simulink model "pid_2"  (Simulink 8.3)
settings: Solver=ode45  StartTime=0.0  StopTime=15  RelTol=1e-3
values from neighbouring files (symbols this model uses):
  Kc = (1.2*tau)/(K*td)    [pid2.m]    (also in pid2.mat = 2.07538801239)
  Kc1 = 0.33*Ku    [pid2.m]    (also in pid2.mat = 3.52049795251)
  Td = 0.5*td    [pid2.m]    (also in pid2.mat = 0.341127043943)
  Td1 = 0.333*Tu    [pid2.m]    (also in pid2.mat = 0.603957217903)
  Ti = 2*td    [pid2.m]    (also in pid2.mat = 1.36450817577)
  Ti1 = 0.5*Tu    [pid2.m]    (also in pid2.mat = 0.906842669523)
libraries: simulink x1
settings Model: Creator=IvanBurgos  LastModifiedBy=IvanBurgos
settings DataIOCC: SignalLoggingSaveFormat=Dataset
settings DebuggingCC: UnderspecifiedInitializationDetection=Simplified  StateNameClashWarn=none
settings GRTTargetCC: CombineOutputUpdateFcns=on  GRTInterface=off

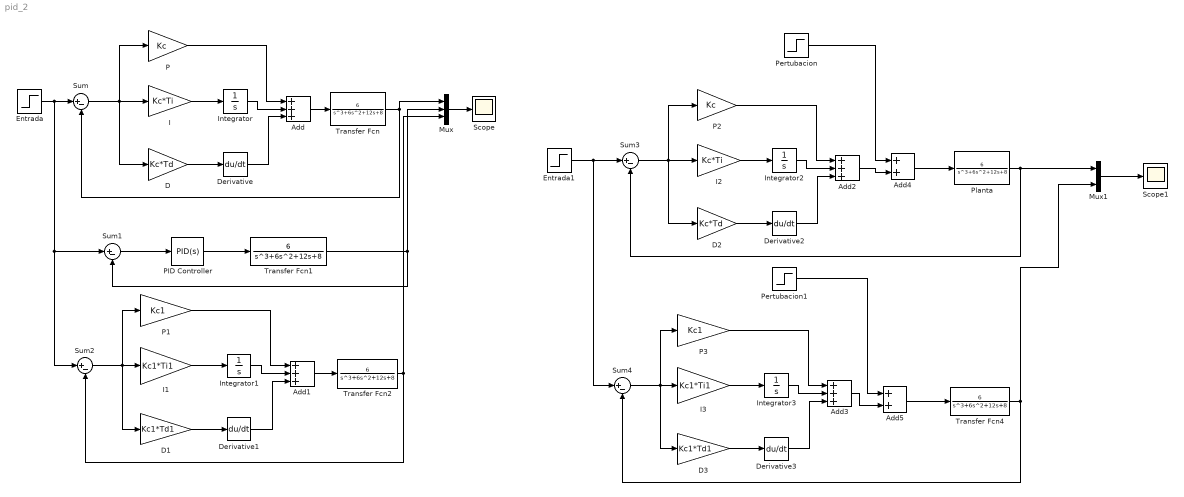
== system pid_2 ==
  Add{,1..3} (4 alike) : Sum  Inputs=+++
  Add4 : Sum
  Add5 : Sum
  D : Gain  Gain=Kc*Td
  D1 : Gain  Gain=Kc1*Td1
  D2 : Gain  Gain=Kc*Td
  D3 : Gain  Gain=Kc1*Td1
  Derivative{,1..3} (4 alike) : Derivative
  Entrada : Step  SampleTime=0
  Entrada1 : Step  SampleTime=0
  I : Gain  Gain=Kc*Ti
  I1 : Gain  Gain=Kc1*Ti1
  I2 : Gain  Gain=Kc*Ti
  I3 : Gain  Gain=Kc1*Ti1
  Integrator{,1..3} (4 alike) : Integrator
  Mux : Mux  Inputs=3
  Mux1 : Mux  Inputs=2
  P : Gain  Gain=Kc
  P1 : Gain  Gain=Kc1
  P2 : Gain  Gain=Kc
  P3 : Gain  Gain=Kc1
  PID Controller : simulink/Continuous/PID Controller  Controller=PID  TimeDomain=Continuous-time  SampleTime=1  IntegratorMethod=Forward Euler  FilterMethod=Forward Euler  Form=Parallel  P=2.01609583089687  I=1.55701135044982  D=0.591682602009288  N=136.60149932365  InitialConditionSource=internal  InitialConditionForIntegrator=0  InitialConditionForFilter=0  ExternalReset=none  LimitOutput=off  UpperSaturationLimit=inf  LowerSaturationLimit=-inf  LinearizeAsGain=on  AntiWindupMode=none  Kb=1  TrackingMode=off  Kt=1  PParamMin=[]  PParamMax=[]  IParamMin=[]  IParamMax=[]  DParamMin=[]  DParamMax=[]  NParamMin=[]  NParamMax=[]  KbParamMin=[]  KbParamMax=[]  KtParamMin=[]  KtParamMax=[]  POutMin=[]  POutMax=[]  IOutMin=[]  IOutMax=[]  DOutMin=[]  DOutMax=[]  NOutMin=[]  NOutMax=[]  KbOutMin=[]  KbOutMax=[]  KtOutMin=[]  KtOutMax=[]  IntegratorOutMin=[]  IntegratorOutMax=[]  FilterOutMin=[]  FilterOutMax=[]  SumOutMin=[]  SumOutMax=[]  SumI1OutMin=[]  SumI1OutMax=[]  SumI2OutMin=[]  SumI2OutMax=[]  SumI3OutMin=[]  SumI3OutMax=[]  SumDOutMin=[]  SumDOutMax=[]  SaturationOutMin=[]  SaturationOutMax=[]  IntegratorContinuousStateAttributes=''  IntegratorStateMustResolveToSignalObject=off  IntegratorRTWStateStorageClass=Auto  FilterContinuousStateAttributes=''  FilterStateMustResolveToSignalObject=off  FilterRTWStateStorageClass=Auto
  Pertubacion : Step  Time=10  SampleTime=0
  Pertubacion1 : Step  Time=10  SampleTime=0
  Planta : TransferFcn  Numerator=[6]  Denominator=[1 6 12 8]
  Scope : Scope
  Scope1 : Scope
  Sum{,1..4} (5 alike) : Sum  Inputs=|+-
  Transfer Fcn{,1..2,4} (4 alike) : TransferFcn  Numerator=[6]  Denominator=[1 6 12 8]
  wires:
  Entrada/1 -> Sum2/1, Sum1/1, Sum/1
  Sum/1 -> D/1, I/1, P/1
  P/1 -> Add/1
  I/1 -> Integrator/1
  Integrator/1 -> Add/2
  Derivative/1 -> Add/3
  D/1 -> Derivative/1
  Add/1 -> Transfer Fcn/1
  Transfer Fcn/1 -> Sum/2, Mux/1
  PID Controller/1 -> Transfer Fcn1/1
  Transfer Fcn1/1 -> Sum1/2, Mux/2
  Mux/1 -> Scope/1
  Sum1/1 -> PID Controller/1
  Sum2/1 -> D1/1, I1/1, P1/1
  P1/1 -> Add1/1
  I1/1 -> Integrator1/1
  Integrator1/1 -> Add1/2
  Derivative1/1 -> Add1/3
  D1/1 -> Derivative1/1
  Add1/1 -> Transfer Fcn2/1
  Transfer Fcn2/1 -> Mux/3, Sum2/2
  Sum3/1 -> D2/1, I2/1, P2/1
  P2/1 -> Add2/1
  I2/1 -> Integrator2/1
  Integrator2/1 -> Add2/2
  Derivative2/1 -> Add2/3
  D2/1 -> Derivative2/1
  Planta/1 -> Mux1/1, Sum3/2
  Sum4/1 -> D3/1, I3/1, P3/1
  P3/1 -> Add3/1
  I3/1 -> Integrator3/1
  Integrator3/1 -> Add3/2
  Derivative3/1 -> Add3/3
  D3/1 -> Derivative3/1
  Transfer Fcn4/1 -> Sum4/2, Mux1/2
  Entrada1/1 -> Sum4/1, Sum3/1
  Pertubacion/1 -> Add4/1
  Add2/1 -> Add4/2
  Add4/1 -> Planta/1
  Pertubacion1/1 -> Add5/1
  Add3/1 -> Add5/2
  Add5/1 -> Transfer Fcn4/1
  Mux1/1 -> Scope1/1
